simulink model "SC_FFNN_trainlm_15_15_15_15_Dec_8_M"  (R2021a)
settings: Solver=VariableStepAuto  StartTime=0.0  StopTime=35  FixedStep=0.1  MaxStep=.1  RelTol=1e-3
model workspace (MAT data in the model file):
  T = [0 0.05 0.1 0.15 0.2 0.25 0.3 0.35 0.4 0.45 0.5 0.55 ... (701 elements, 701x1)]
  U = [3.99594136536 3.99594136536 3.99594136536 3.99594136536 3.99594136536 3.99594136536 3.99594136536 3.99594136536 3.99594136536 3.99594136536 3.99594136536 3.99594136536 ... (701 elements, 701x1)]
libraries: neural x66, simulink_extras x2
(part 3 of 3)

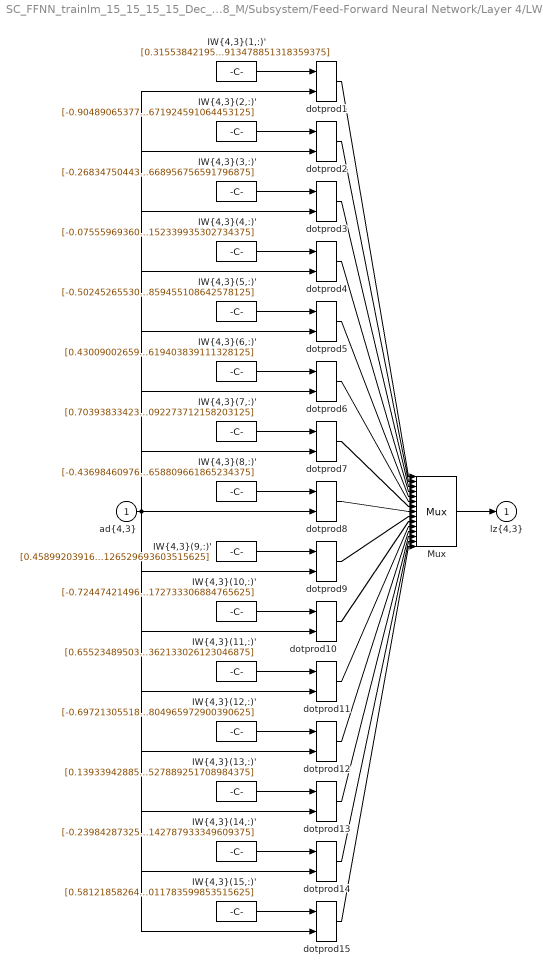
== system SC_FFNN_trainlm_15_15_15_15_Dec_8_M/Subsystem/Feed-Forward Neural Network/Layer 4/LW{4,3} ==
  "ad{4,3}" : Inport  PortDimensions=15
      mask Display: e = 0.06;c1 = [120 230 180]/255;c2 = ([120 230 180]+0)/(256+128);c3 = ([120 230 180]+128)/(256+128);patch([0 1 1 0],[0 0 1 1],c1);patch([0 1 1 1-e 1-e 0+e],[0 0 1 1-e 0+e 0+e],c2);patch([0 0 1 1-e 0+e 0+e],[0 1 1 1-e 1-e 0+e],c3);plot([0 1 1 0 0],[0 0 1 1 0]);
  "IW{4,3}(1,:)'" : Constant  Value=[0.31553842195222447930547104988363571465015411376953125;0.0075615715523118520735579295433126389980316162109375;-0.94721511754231624280464529874734580516815185546875;0.85481367567669208629155264134169556200504302978515625;0.75380956202653182085526850642054341733455657958984375;0.0077755469209772609673336773994378745555877685546875;-0.429675723526083519487883677356876432895660400390625;0.667590670480306069833886795095168054103851318359375;0.51860039974835803189279204161721281707286834716796875;-0.08373192794011165285272824121420853771269321441650390625;-0.2175362396201991621591531611557002179324626922607421875;-0.7659263609886843848784110377891920506954193115234375;0.65482216980151275453891912547987885773181915283203125;1.0011468332773805212099205164122395217418670654296875;0.84432973040632131045413188985548913478851318359375]
      mask Display: e = 0.06;c1 = [120 150 230]/255;c2 = ([120 150 230]+0)/383;c3 = ([120 150 230]+128)/383;patch([0 1 1 0],[0 0 1 1],c1);patch([0 1 1 1-e 1-e 0+e],[0 0 1 1-e 0+e 0+e],c2);patch([0 0 1 1-e 0+e 0+e],[0 1 1 1-e 1-e 0+e],c3);plot([0 1 1 0 0],[0 0 1 1 0]);disp('weights');
  "IW{4,3}(10,:)'" : Constant  Value=[-0.7244742149609673109722507433616556227207183837890625;0.334240600080149885542368792812339961528778076171875;-0.28139807062526023262449825779185630381107330322265625;-0.8904164201605351269819266235572285950183868408203125;0.606728251104347027222729593631811439990997314453125;-0.732992280677375429576159149291925132274627685546875;-0.78155895308659584230781547375954687595367431640625;-0.894626873075079487307448289357125759124755859375;0.68377563973833754840114806938800029456615447998046875;-0.3448488302893306656216054761898703873157501220703125;0.7688100905519898997653172045829705893993377685546875;-0.2037382409373282854403441888280212879180908203125;-0.706295634632664093288667572778649628162384033203125;-0.16190860431920028883467921332339756190776824951171875;-0.489763083180007774419806310106650926172733306884765625]
      mask Display: e = 0.06;c1 = [120 150 230]/255;c2 = ([120 150 230]+0)/383;c3 = ([120 150 230]+128)/383;patch([0 1 1 0],[0 0 1 1],c1);patch([0 1 1 1-e 1-e 0+e],[0 0 1 1-e 0+e 0+e],c2);patch([0 0 1 1-e 0+e 0+e],[0 1 1 1-e 1-e 0+e],c3);plot([0 1 1 0 0],[0 0 1 1 0]);disp('weights');
  "IW{4,3}(11,:)'" : Constant  Value=[0.655234895033436348654731773422099649906158447265625;0.172879229357835839664403465576469898223876953125;-0.6667947658530162247103589834296144545078277587890625;-0.403369405118854162939356911010690964758396148681640625;-0.1318544828545334113290010691343923099339008331298828125;-0.9568882255930060143356286062044091522693634033203125;-0.106920408301278413443213821665267460048198699951171875;-0.1867584040453882099352966861260938458144664764404296875;0.8090732204259529769529990517185069620609283447265625;-0.441789763295113602215025139230419881641864776611328125;0.4417113416338629416912908709491603076457977294921875;0.03073443842314471652343854657374322414398193359375;-0.70967334776365731396907676753471605479717254638671875;0.64618117704675637202882398923975415527820587158203125;-0.10484948585139435006663433114226791076362133026123046875]
      mask Display: e = 0.06;c1 = [120 150 230]/255;c2 = ([120 150 230]+0)/383;c3 = ([120 150 230]+128)/383;patch([0 1 1 0],[0 0 1 1],c1);patch([0 1 1 1-e 1-e 0+e],[0 0 1 1-e 0+e 0+e],c2);patch([0 0 1 1-e 0+e 0+e],[0 1 1 1-e 1-e 0+e],c3);plot([0 1 1 0 0],[0 0 1 1 0]);disp('weights');
  "IW{4,3}(12,:)'" : Constant  Value=[-0.697213055181517216141173776122741401195526123046875;0.3502248328102306462739079506718553602695465087890625;-0.50701362367857527591041844061692245304584503173828125;-0.952933150655576266530033535673283040523529052734375;-0.142730264666183381816466635427786968648433685302734375;0.11968141174501933932106112479232251644134521484375;0.164693067035057427727195999977993778884410858154296875;0.425751029033640315812903054393245838582515716552734375;0.23896595861192981846699012749013490974903106689453125;0.59750557167956330761882099977810867130756378173828125;-0.96277456469693445395563458077958784997463226318359375;0.315061084191821993982784988475032150745391845703125;0.08703130986387407064253096677930443547666072845458984375;-0.1876204978432067793647775033605284988880157470703125;-0.1439042020852066006142422338598407804965972900390625]
      mask Display: e = 0.06;c1 = [120 150 230]/255;c2 = ([120 150 230]+0)/383;c3 = ([120 150 230]+128)/383;patch([0 1 1 0],[0 0 1 1],c1);patch([0 1 1 1-e 1-e 0+e],[0 0 1 1-e 0+e 0+e],c2);patch([0 0 1 1-e 0+e 0+e],[0 1 1 1-e 1-e 0+e],c3);plot([0 1 1 0 0],[0 0 1 1 0]);disp('weights');
  "IW{4,3}(13,:)'" : Constant  Value=[0.1393394288591347784933560660647344775497913360595703125;-0.2779559016106782909361072597675956785678863525390625;-0.3793105443459456882493441298720426857471466064453125;-0.561286457886370993008995355921797454357147216796875;0.115142610227820352264416214893572032451629638671875;-0.3983619638610218505192506199819035828113555908203125;0.07249072952965031346739266382428468205034732818603515625;0.8674513190918593519285195725387893617153167724609375;0.1901645443965586934620404235829482786357402801513671875;-0.21658047074431963086027508325059898197650909423828125;0.407767224123357141518653179446118883788585662841796875;0.9018303965299183655446313423453830182552337646484375;0.7221593924901472671962210370111279189586639404296875;0.190306601081223103477668701088987290859222412109375;0.944173407450308754818024681298993527889251708984375]
      mask Display: e = 0.06;c1 = [120 150 230]/255;c2 = ([120 150 230]+0)/383;c3 = ([120 150 230]+128)/383;patch([0 1 1 0],[0 0 1 1],c1);patch([0 1 1 1-e 1-e 0+e],[0 0 1 1-e 0+e 0+e],c2);patch([0 0 1 1-e 0+e 0+e],[0 1 1 1-e 1-e 0+e],c3);plot([0 1 1 0 0],[0 0 1 1 0]);disp('weights');
  "IW{4,3}(14,:)'" : Constant  Value=[-0.2398428732506267813118228104940499179065227508544921875;0.24055685414217098383460324839688837528228759765625;0.5556503204465510492582325241528451442718505859375;0.400224819084944616331966926736640743911266326904296875;-0.514215186761521891867232625372707843780517578125;0.878819427746916570498569853953085839748382568359375;-0.39014020012771533085782493799342773854732513427734375;0.70763972547696385451132528032758273184299468994140625;-0.8074554095311119450428805066621862351894378662109375;0.79276908126501288709420123268500901758670806884765625;-0.1777740947523782921724233574423124082386493682861328125;0.444697028654995829555218733730725944042205810546875;0.80605329656889612710557457830873318016529083251953125;0.62356546006238711132851904039853252470493316650390625;0.2139428087530726718679119358057505451142787933349609375]
      mask Display: e = 0.06;c1 = [120 150 230]/255;c2 = ([120 150 230]+0)/383;c3 = ([120 150 230]+128)/383;patch([0 1 1 0],[0 0 1 1],c1);patch([0 1 1 1-e 1-e 0+e],[0 0 1 1-e 0+e 0+e],c2);patch([0 0 1 1-e 0+e 0+e],[0 1 1 1-e 1-e 0+e],c3);plot([0 1 1 0 0],[0 0 1 1 0]);disp('weights');
  "IW{4,3}(15,:)'" : Constant  Value=[0.5812185826402129773526894496171735227108001708984375;0.6223017702005704254730744651169516146183013916015625;-0.493328121690028431611807491208310239017009735107421875;0.5026308266314780670569462017738260328769683837890625;0.61199352026972253515424426950630731880664825439453125;0.961807272093718079730706449481658637523651123046875;1.046151678134404239273180792224593460559844970703125;-0.147295039259621785010523353776079602539539337158203125;1.0063463316647920375856983810081146657466888427734375;0.64319939559936722961452915114932693541049957275390625;-0.03390297909234755990848242390711675398051738739013671875;-0.1998405092753248180059699734556488692760467529296875;0.33725469223986304090345811346196569502353668212890625;0.79956904751505331052641167843830771744251251220703125;0.4139034664216669767711209715344011783599853515625]
      mask Display: e = 0.06;c1 = [120 150 230]/255;c2 = ([120 150 230]+0)/383;c3 = ([120 150 230]+128)/383;patch([0 1 1 0],[0 0 1 1],c1);patch([0 1 1 1-e 1-e 0+e],[0 0 1 1-e 0+e 0+e],c2);patch([0 0 1 1-e 0+e 0+e],[0 1 1 1-e 1-e 0+e],c3);plot([0 1 1 0 0],[0 0 1 1 0]);disp('weights');
  "IW{4,3}(2,:)'" : Constant  Value=[-0.904890653772267850030175395659171044826507568359375;-0.0208113225532915446791548674809746444225311279296875;-0.8322529834342002885705369408242404460906982421875;-0.201960061930889001047262354404665529727935791015625;0.1648659289748206635550786813837476074695587158203125;0.293619332545560940417317397077567875385284423828125;0.601640573903069242334140653838403522968292236328125;0.698170959908910315760977027821354568004608154296875;-0.1659050925144660570964560974971391260623931884765625;-0.5886553210720730788807486533187329769134521484375;-0.004194114071626842132900492288172245025634765625;0.629363379037164438756235540495254099369049072265625;-0.7313233165425836457274044732912443578243255615234375;0.1070831469910651367882792328600771725177764892578125;-0.61843070398175559176934257266111671924591064453125]
      mask Display: e = 0.06;c1 = [120 150 230]/255;c2 = ([120 150 230]+0)/383;c3 = ([120 150 230]+128)/383;patch([0 1 1 0],[0 0 1 1],c1);patch([0 1 1 1-e 1-e 0+e],[0 0 1 1-e 0+e 0+e],c2);patch([0 0 1 1-e 0+e 0+e],[0 1 1 1-e 1-e 0+e],c3);plot([0 1 1 0 0],[0 0 1 1 0]);disp('weights');
  "IW{4,3}(3,:)'" : Constant  Value=[-0.268347504432777383964747741629253141582012176513671875;0.754097446770087831424689284176565706729888916015625;0.75263874515231499184864105700398795306682586669921875;-0.901842802270846899403977658948861062526702880859375;-0.9099732739126566993803635341464541852474212646484375;-0.384508835938118576081024002633057534694671630859375;0.78318313263372763000091936191893182694911956787109375;-0.15005450935687070224133776719099842011928558349609375;1.0353563189562862145720600892673246562480926513671875;0.8119656783224875606919113124604336917400360107421875;0.386306816916898776437250262461020611226558685302734375;-0.3502891227389819395199310747557319700717926025390625;-0.833925762881452481423139033722691237926483154296875;0.1208430471852764143125824602975626476109027862548828125;-0.354436614484288259330213577413815073668956756591796875]
      mask Display: e = 0.06;c1 = [120 150 230]/255;c2 = ([120 150 230]+0)/383;c3 = ([120 150 230]+128)/383;patch([0 1 1 0],[0 0 1 1],c1);patch([0 1 1 1-e 1-e 0+e],[0 0 1 1-e 0+e 0+e],c2);patch([0 0 1 1-e 0+e 0+e],[0 1 1 1-e 1-e 0+e],c3);plot([0 1 1 0 0],[0 0 1 1 0]);disp('weights');
  "IW{4,3}(4,:)'" : Constant  Value=[-0.075559693607434808004796877867192961275577545166015625;-0.2937163741220889523475534588214941322803497314453125;0.140782807194338610567996283862157724797725677490234375;-0.327512148065631725213364688897854648530483245849609375;0.79690181259091763532609320463961921632289886474609375;-0.7225507278437108826807389050372876226902008056640625;0.1606545464276571688611028321247431449592113494873046875;0.278892264121990807179685134542523883283138275146484375;0.99879009005094865347729182758484967052936553955078125;0.48887017369220508999916319226031191647052764892578125;0.6299850656391872139039378453162498772144317626953125;-0.507543771530717169326862858724780380725860595703125;-0.80998120590582678435254138094023801386356353759765625;-0.27568122676592532460659867865615524351596832275390625;0.85726622960898646308436354956938885152339935302734375]
      mask Display: e = 0.06;c1 = [120 150 230]/255;c2 = ([120 150 230]+0)/383;c3 = ([120 150 230]+128)/383;patch([0 1 1 0],[0 0 1 1],c1);patch([0 1 1 1-e 1-e 0+e],[0 0 1 1-e 0+e 0+e],c2);patch([0 0 1 1-e 0+e 0+e],[0 1 1 1-e 1-e 0+e],c3);plot([0 1 1 0 0],[0 0 1 1 0]);disp('weights');
  "IW{4,3}(5,:)'" : Constant  Value=[-0.50245265530528182562619576856377534568309783935546875;-0.1011128868565034366611143923364579677581787109375;-0.689020855120729525111755719990469515323638916015625;0.443731904654277753419222563024959526956081390380859375;0.54225389484726049804663716713548637926578521728515625;-0.04885413240487412878110262681730091571807861328125;0.784584663933904469246272128657437860965728759765625;0.8078184438938382783135239151306450366973876953125;0.776557734583537051520352179068140685558319091796875;0.73149167656120628322469201521016657352447509765625;0.170333901432133671960400533862411975860595703125;-0.31457355775344097992274328134953975677490234375;-0.597515228487570215776258919504471123218536376953125;-0.031886165259437750096882524530883529223501682281494140625;0.264904332519398544310007537205819971859455108642578125]
      mask Display: e = 0.06;c1 = [120 150 230]/255;c2 = ([120 150 230]+0)/383;c3 = ([120 150 230]+128)/383;patch([0 1 1 0],[0 0 1 1],c1);patch([0 1 1 1-e 1-e 0+e],[0 0 1 1-e 0+e 0+e],c2);patch([0 0 1 1-e 0+e 0+e],[0 1 1 1-e 1-e 0+e],c3);plot([0 1 1 0 0],[0 0 1 1 0]);disp('weights');
  "IW{4,3}(6,:)'" : Constant  Value=[0.430090026592353069645469076931476593017578125;0.9270605736868537949391111396835185587406158447265625;-0.150738275383345499136567013920284807682037353515625;0.59681032440129266891659653992974199354648590087890625;-0.424740295258490885288438221323303878307342529296875;-0.2750814383625079795336887400480918586254119873046875;0.8994617874874879515090242421138100326061248779296875;0.86700321701421056985736868227832019329071044921875;0.00141585204143073795958474025979967336752451956272125244140625;-0.42892626844830872290259549117763526737689971923828125;0.2039859881032530797284607615438289940357208251953125;-0.24861571998082343526448312331922352313995361328125;-0.398234926141676937039193262535263784229755401611328125;-0.10913571888412824939518230848989333026111125946044921875;0.07443230778754945931030562178420950658619403839111328125]
      mask Display: e = 0.06;c1 = [120 150 230]/255;c2 = ([120 150 230]+0)/383;c3 = ([120 150 230]+128)/383;patch([0 1 1 0],[0 0 1 1],c1);patch([0 1 1 1-e 1-e 0+e],[0 0 1 1-e 0+e 0+e],c2);patch([0 0 1 1-e 0+e 0+e],[0 1 1 1-e 1-e 0+e],c3);plot([0 1 1 0 0],[0 0 1 1 0]);disp('weights');
  "IW{4,3}(7,:)'" : Constant  Value=[0.703938334239562646388321809354238212108612060546875;-0.9154044041709143986196295372792519629001617431640625;-0.71674676776983214931959764726343564689159393310546875;0.0898117964893430098527460359036922454833984375;0.0902527291814633481070728748818510212004184722900390625;0.5762268567970945110090497109922580420970916748046875;0.11853881328069211520404024895469774492084980010986328125;0.317823384137706776986220802427851594984531402587890625;-0.2224855726601190630820070737172500230371952056884765625;0.1734865814491053648271901010957662947475910186767578125;-0.3479156581544173842956979569862596690654754638671875;0.093107586165917854970075495657511055469512939453125;-0.409571879764876134455420242375112138688564300537109375;-0.90080881304685955779376627106103114783763885498046875;0.2076805817685472288491865811010939069092273712158203125]
      mask Display: e = 0.06;c1 = [120 150 230]/255;c2 = ([120 150 230]+0)/383;c3 = ([120 150 230]+128)/383;patch([0 1 1 0],[0 0 1 1],c1);patch([0 1 1 1-e 1-e 0+e],[0 0 1 1-e 0+e 0+e],c2);patch([0 0 1 1-e 0+e 0+e],[0 1 1 1-e 1-e 0+e],c3);plot([0 1 1 0 0],[0 0 1 1 0]);disp('weights');
  "IW{4,3}(8,:)'" : Constant  Value=[-0.4369846097628933279111151932738721370697021484375;0.945916668281269412688061493099667131900787353515625;-0.4631223572054337100922793979407288134098052978515625;0.372529313530939598653191069388412870466709136962890625;0.968501557071904439766285577206872403621673583984375;0.5605916416882192887527480706921778619289398193359375;0.415055353336941490471900806369376368820667266845703125;-0.58644708412978996392439512419514358043670654296875;-0.589502508512038669863386530778370797634124755859375;0.2507988186648664186151336252805776894092559814453125;-0.087150798296506071238809454371221363544464111328125;0.1238403085319534913111283458420075476169586181640625;-1.0297496221689323991910214317613281309604644775390625;0.736517215060549457206207080162130296230316162109375;0.6037764076624492215472628231509588658809661865234375]
      mask Display: e = 0.06;c1 = [120 150 230]/255;c2 = ([120 150 230]+0)/383;c3 = ([120 150 230]+128)/383;patch([0 1 1 0],[0 0 1 1],c1);patch([0 1 1 1-e 1-e 0+e],[0 0 1 1-e 0+e 0+e],c2);patch([0 0 1 1-e 0+e 0+e],[0 1 1 1-e 1-e 0+e],c3);plot([0 1 1 0 0],[0 0 1 1 0]);disp('weights');
  "IW{4,3}(9,:)'" : Constant  Value=[0.458992039160482645510086285867146216332912445068359375;-0.6215863137552479766867463695234619081020355224609375;-0.473171431126564179248106256636674515902996063232421875;0.7835775006121619146171042302739806473255157470703125;0.435303850481669696304010130916140042245388031005859375;0.33702442850708980159879502025432884693145751953125;0.1446448833036879932922857960875262506306171417236328125;0.30770118412517621919732846436090767383575439453125;0.59630358841047215179287377395667135715484619140625;-0.6779993046408103740674278014921583235263824462890625;0.44992460630928132747641257083159871399402618408203125;-0.20835554275199807960916587035171687602996826171875;0.042725944984608597854158773543531424365937709808349609375;-0.8955605394963199739066794791142456233501434326171875;0.042460118816029103483433715382489026524126529693603515625]
      mask Display: e = 0.06;c1 = [120 150 230]/255;c2 = ([120 150 230]+0)/383;c3 = ([120 150 230]+128)/383;patch([0 1 1 0],[0 0 1 1],c1);patch([0 1 1 1-e 1-e 0+e],[0 0 1 1-e 0+e 0+e],c2);patch([0 0 1 1-e 0+e 0+e],[0 1 1 1-e 1-e 0+e],c3);plot([0 1 1 0 0],[0 0 1 1 0]);disp('weights');
  Mux : Mux  Inputs=15
      mask Display: e = 0.06;c1 = [120 150 230]/255;c2 = ([120 150 230]+0)/383;c3 = ([120 150 230]+128)/383;patch([0 1 1 0],[0 0 1 1],c1);patch([0 1 1 1-e 1-e 0+e],[0 0 1 1-e 0+e 0+e],c2);patch([0 0 1 1-e 0+e 0+e],[0 1 1 1-e 1-e 0+e],c3);plot([0 1 1 0 0],[0 0 1 1 0]);disp('Mux');
  dotprod{1..15} (15 alike) : neural/Weight Functions/dotprod
  "lz{4,3}" : Outport
      mask Display: e = 0.06;c1 = [120 230 180]/255;c2 = ([120 230 180]+0)/(256+128);c3 = ([120 230 180]+128)/(256+128);patch([0 1 1 0],[0 0 1 1],c1);patch([0 1 1 1-e 1-e 0+e],[0 0 1 1-e 0+e 0+e],c2);patch([0 0 1 1-e 0+e 0+e],[0 1 1 1-e 1-e 0+e],c3);plot([0 1 1 0 0],[0 0 1 1 0]);
  wires:
  "IW{4,3}(1,:)'"/1 -> dotprod1/1
  "ad{4,3}"/1 -> dotprod1/2, dotprod2/2, dotprod3/2, dotprod4/2, dotprod5/2, dotprod6/2, dotprod7/2, dotprod8/2, dotprod9/2, dotprod10/2, dotprod11/2, dotprod12/2, dotprod13/2, dotprod14/2, dotprod15/2
  dotprod1/1 -> Mux/1
  "IW{4,3}(2,:)'"/1 -> dotprod2/1
  dotprod2/1 -> Mux/2
  "IW{4,3}(3,:)'"/1 -> dotprod3/1
  dotprod3/1 -> Mux/3
  "IW{4,3}(4,:)'"/1 -> dotprod4/1
  dotprod4/1 -> Mux/4
  "IW{4,3}(5,:)'"/1 -> dotprod5/1
  dotprod5/1 -> Mux/5
  "IW{4,3}(6,:)'"/1 -> dotprod6/1
  dotprod6/1 -> Mux/6
  "IW{4,3}(7,:)'"/1 -> dotprod7/1
  dotprod7/1 -> Mux/7
  "IW{4,3}(8,:)'"/1 -> dotprod8/1
  dotprod8/1 -> Mux/8
  "IW{4,3}(9,:)'"/1 -> dotprod9/1
  dotprod9/1 -> Mux/9
  "IW{4,3}(10,:)'"/1 -> dotprod10/1
  dotprod10/1 -> Mux/10
  "IW{4,3}(11,:)'"/1 -> dotprod11/1
  dotprod11/1 -> Mux/11
  "IW{4,3}(12,:)'"/1 -> dotprod12/1
  dotprod12/1 -> Mux/12
  "IW{4,3}(13,:)'"/1 -> dotprod13/1
  dotprod13/1 -> Mux/13
  "IW{4,3}(14,:)'"/1 -> dotprod14/1
  dotprod14/1 -> Mux/14
  "IW{4,3}(15,:)'"/1 -> dotprod15/1
  dotprod15/1 -> Mux/15
  Mux/1 -> "lz{4,3}"/1

== system SC_FFNN_trainlm_15_15_15_15_Dec_8_M/Subsystem/Feed-Forward Neural Network/Layer 5/Delays 1 ==
  "p{5}" : Inport  PortDimensions=15
      mask Display: e = 0.06;c1 = [120 230 180]/255;c2 = ([120 230 180]+0)/(256+128);c3 = ([120 230 180]+128)/(256+128);patch([0 1 1 0],[0 0 1 1],c1);patch([0 1 1 1-e 1-e 0+e],[0 0 1 1-e 0+e 0+e],c2);patch([0 0 1 1-e 0+e 0+e],[0 1 1 1-e 1-e 0+e],c3);plot([0 1 1 0 0],[0 0 1 1 0]);
  mux : Mux  Inputs=1
      mask Display: e = 0.06;c1 = [120 150 230]/255;c2 = ([120 150 230]+0)/383;c3 = ([120 150 230]+128)/383;patch([0 1 1 0],[0 0 1 1],c1);patch([0 1 1 1-e 1-e 0+e],[0 0 1 1-e 0+e 0+e],c2);patch([0 0 1 1-e 0+e 0+e],[0 1 1 1-e 1-e 0+e],c3);plot([0 1 1 0 0],[0 0 1 1 0]);disp('Mux')
  "pd{5,4}" : Outport
      mask Display: e = 0.06;c1 = [120 230 180]/255;c2 = ([120 230 180]+0)/(256+128);c3 = ([120 230 180]+128)/(256+128);patch([0 1 1 0],[0 0 1 1],c1);patch([0 1 1 1-e 1-e 0+e],[0 0 1 1-e 0+e 0+e],c2);patch([0 0 1 1-e 0+e 0+e],[0 1 1 1-e 1-e 0+e],c3);plot([0 1 1 0 0],[0 0 1 1 0]);
  wires:
  "p{5}"/1 -> mux/1
  mux/1 -> "pd{5,4}"/1

== system SC_FFNN_trainlm_15_15_15_15_Dec_8_M/Subsystem/Feed-Forward Neural Network/Layer 5/LW{5,4} ==
  "ad{5,4}" : Inport  PortDimensions=15
      mask Display: e = 0.06;c1 = [120 230 180]/255;c2 = ([120 230 180]+0)/(256+128);c3 = ([120 230 180]+128)/(256+128);patch([0 1 1 0],[0 0 1 1],c1);patch([0 1 1 1-e 1-e 0+e],[0 0 1 1-e 0+e 0+e],c2);patch([0 0 1 1-e 0+e 0+e],[0 1 1 1-e 1-e 0+e],c3);plot([0 1 1 0 0],[0 0 1 1 0]);
  "IW{5,4}(1,:)'" : Constant  Value=[-0.05023486315304752369836904790645348839461803436279296875;0.387505148267826893260235010529868304729461669921875;0.70749468870990261937237164602265693247318267822265625;0.4193877940677595006491173990070819854736328125;0.55021103217860345413470213316031731665134429931640625;-0.732841924312341408409565701731480658054351806640625;-0.09359170492947703479114096580815385095775127410888671875;0.1904292647133191407338159706341684795916080474853515625;-0.11755289898159253236809007603369536809623241424560546875;-0.429261035730314655101125254077487625181674957275390625;-0.45884687071140695113768970259116031229496002197265625;0.8707043402672558496391275184578262269496917724609375;-0.6239652323667181921251767562353052198886871337890625;0.57396316356903664956945476660621352493762969970703125;-1.050933724631924359727008777554146945476531982421875]
      mask Display: e = 0.06;c1 = [120 150 230]/255;c2 = ([120 150 230]+0)/383;c3 = ([120 150 230]+128)/383;patch([0 1 1 0],[0 0 1 1],c1);patch([0 1 1 1-e 1-e 0+e],[0 0 1 1-e 0+e 0+e],c2);patch([0 0 1 1-e 0+e 0+e],[0 1 1 1-e 1-e 0+e],c3);plot([0 1 1 0 0],[0 0 1 1 0]);disp('weights');
  Mux : Mux  Inputs=1
      mask Display: e = 0.06;c1 = [120 150 230]/255;c2 = ([120 150 230]+0)/383;c3 = ([120 150 230]+128)/383;patch([0 1 1 0],[0 0 1 1],c1);patch([0 1 1 1-e 1-e 0+e],[0 0 1 1-e 0+e 0+e],c2);patch([0 0 1 1-e 0+e 0+e],[0 1 1 1-e 1-e 0+e],c3);plot([0 1 1 0 0],[0 0 1 1 0]);disp('Mux');
  dotprod1 : neural/Weight Functions/dotprod
  "lz{5,4}" : Outport
      mask Display: e = 0.06;c1 = [120 230 180]/255;c2 = ([120 230 180]+0)/(256+128);c3 = ([120 230 180]+128)/(256+128);patch([0 1 1 0],[0 0 1 1],c1);patch([0 1 1 1-e 1-e 0+e],[0 0 1 1-e 0+e 0+e],c2);patch([0 0 1 1-e 0+e 0+e],[0 1 1 1-e 1-e 0+e],c3);plot([0 1 1 0 0],[0 0 1 1 0]);
  wires:
  "IW{5,4}(1,:)'"/1 -> dotprod1/1
  "ad{5,4}"/1 -> dotprod1/2
  dotprod1/1 -> Mux/1
  Mux/1 -> "lz{5,4}"/1
